simulink model "ModelPlant_DP_v3"  (R2015a)
settings: Solver=ode3  StartTime=0.0  StopTime=Simulation_Time  FixedStep=0.01  RelTol=1e-3
values from neighbouring files (symbols this model uses):
  DesiredPath = 0    [Innput.m]    (also in Input_v3.m = 1)
  Elipscenter_radi = [6 5;0 3 ]    [Innput.m]    (also in Input_v3.m)
  eta_dot_ini = [7;0;0]    [Innput.m]    (also in Input_v3.m)
  K = [2;10]    [Input_v3.m]
  K1 = diag([1,1,4])    [Input_v3.m]
  K2 = diag([200,50,3])    [Input_v3.m]    (also in inputDPgains.m = [1 0 0; 0 1 0; 0 0 1])
  l1 = [1 0 0;0 1 0;0 0 0.05]    [Input_v3.m]    (also in inputDPgains.m = [1 0 0; 0 1 0; 0 0 0.05])
  l2 = [1 0 0;0 1 0;0 0 0.05]    [Input_v3.m]    (also in inputDPgains.m = [1 0 0; 0 1 0; 0 0 0.05])
  l3 = [1 0 0;0 1 0;0 0 0.05]    [Input_v3.m]    (also in inputDPgains.m = [1 0 0; 0 1 0; 0 0 0.05])
  L_1 = 0.1    [Input_v3.m]
  L_2 = 2    [Input_v3.m]
  L_3 = 0.01    [Input_v3.m]
  LAW = 1    [Innput.m]    (also in Input_v3.m = 0)
  lim = [1.00;-20;6.45/2;-6.45/2]    [Innput.m]    (also in Input_v3.m = [20;-20;9;-9])
  lim_2 = [1.5;-22;7;-7]    [Innput.m]    (also in Input_v3.m = [25;-25;10;-10])
  m = 14.79    [Input_v3.m]    (also in ctrl_student_init.m)
  mu = mu(1)    [Innput.m]    (also in Input_v3.m = mu(2))
  pd = [2 10;0 4]    [Input_v3.m]
  T_initialDP = T_initialDP*100    (= 0)    [Input_v3.m]
  U_ref = 0.1    [Innput.m]    (also in Input_v3.m)
(part 2 of 2)

== matlab function ModelPlant_DP_v3/Subsystem1/PathParameterization/PathGenerization_Ellips/parameter generator/UpdateLaw ==
  data: s_dot output; p_d_sdot input; U_ref input; U_s output; V_1s input; mu input; eta_ds input; LAW input
function [s_dot,U_s ]= fcn(p_d_sdot,U_ref,V_1s,mu,eta_ds,LAW)


U_s=U_ref/(sqrt(p_d_sdot(1)^2+p_d_sdot(2)^2));
if LAW ==1

        s_dot=U_s-mu*V_1s;
else
        s_dot=U_s-mu/(sqrt(eta_ds(1)^2+eta_ds(2)^2))*V_1s;
end


end

== matlab function ModelPlant_DP_v3/Subsystem1/PathParameterization/PathGenerization_Straight/Path parametization /Subsystem/MATLAB Function ==
  data: InitPosOut output; DesPos input; s_in input; U_ref input; N_iteration input; N_in input; DesPosOut output; SwitchSignal_out output; N_out output; U output; s_out output; Start_time input; init_time output; flag output
function [InitPosOut,DesPosOut,SwitchSignal_out,N_out,U,s_out,init_time,flag]= fcn(DesPos,s_in,U_ref,N_iteration,N_in,Start_time)
[a,b]=size(DesPos);
N_max=b-1;
    init_time=zeros(2,1);
    init_time(1)=Start_time(1)+1;
    init_time(2)=Start_time(2);
   
if flag==2
            N_out=N_in;
            InitPosOut=DesPos(:,N_out);
            DesPosOut=DesPos(:,N_out+1);
            SwitchSignal_out=1;
            s_out=1;
            DP=1;
            flag=2;
else
    
    
if init_time(1)<N_iteration         % DP for N_iterations
    N_out=N_in;
    InitPosOut=DesPos(:,N_out);
    DesPosOut=DesPos(:,N_out+1);
    SwitchSignal_out=1;
    s_out=0;
    DP=1;
    flag=1;
    
else
    if N_in==N_max                  % if we are at final stretch
        if  s_in>=0.9999
            N_out=N_in;
            InitPosOut=DesPos(:,N_out);
            DesPosOut=DesPos(:,N_out+1);
            SwitchSignal_out=1;
            s_out=1;
            DP=1;
            flag=2;
            
        else
            N_out=N_in;
            InitPosOut=DesPos(:,N_in);
            DesPosOut=DesPos(:,N_in+1);
            SwitchSignal_out=1;
            s_out=s_in;
            DP=0;
            flag=3;
            
        end
    else
       if s_in>=0.9999
           if N_in+1 ==N_max
               SwitchSignal_out=0;
               flag=40;
           else
               SwitchSignal_out=0;
               flag=50;
           end
            N_out=N_in+1;
            InitPosOut=DesPos(:,N_out);
            DesPosOut=DesPos(:,N_out+1);
            s_out=1;
            DP=0;

       else 
            if init_time(2)==0;
                init_time(2)=1;
                SwitchSignal_out=0;
                flag=5.75;
            else
                SwitchSignal_out=1;
                flag=5.25;
            end
            N_out=N_in;
            InitPosOut=DesPos(:,N_in);
            DesPosOut=DesPos(:,N_in+1);
            s_out=s_in;
            DP=0;
            
        end
    end
    
end   
if DP==1
    U=0;
else
    U=U_ref*(1.01+ sin(2*pi*s_out-pi/2));
end

end
end

== matlab function ModelPlant_DP_v3/Subsystem1/PathParameterization/PathGenerization_Straight/parameter generator/MATLAB Function1 ==
  data: SwitchSignal_In input; SwitchSignal_Out output
function SwitchSignal_Out = fcn(SwitchSignal_In)

if SwitchSignal_In==0
    SwitchSignal_Out=1;
else
    SwitchSignal_Out=0;
end
    
end

== matlab function ModelPlant_DP_v3/Subsystem1/PathParameterization/PathGenerization_Straight/parameter generator/UpdateLaw ==
  data: s_dot output; p_d_sdot input; U_ref input; U_s output; V_1s input; mu input; eta_ds input; LAW input
function [s_dot,U_s ]= fcn(p_d_sdot,U_ref,V_1s,mu,eta_ds,LAW)


U_s=U_ref/(sqrt(p_d_sdot(1)^2+p_d_sdot(2)^2));
if LAW ==1

        s_dot=U_s-mu*V_1s;
else
        s_dot=U_s-mu/(sqrt(eta_ds(1)^2+eta_ds(2)^2))*V_1s;
end


end

== matlab function ModelPlant_DP_v3/DPObserver1/Bias/bHatDot ==
  data: bHatDot output; L3 input; eta input; etaHat input
function bHatDot = fcn(L3,eta,etaHat)

bHatDot=L3*(eta-etaHat);
%bHatDot=[0;0;0];

end

== matlab function ModelPlant_DP_v3/DPObserver1/D ==
  data: D output; etaHatDot input
function D = fcn(etaHatDot)

u=etaHatDot(1);     %u=0; 
v=etaHatDot(2);     %v=0; 
r=etaHatDot(3);     %r=0;

Xu=-0.6555;
Xuu=0.3545;
Xuuu=-3.787;
Yv=-1.33;
Yvv=-2.776;
Yvvv=-64.91;
Yr=-7.25;
Yrr=-3.45;
Yrrr=0;
Yrv=-0.805;
Yvr=-0.845;
Nv=0;
Nvv=-0.2088;
Nvvv=0;
Nr=-1.9;
Nrr=-0.75;
Nrrr=0;
Nrv=0.13;
Nvr=0.08;

d11=-Xu-Xuu*abs(u)-Xuuu*u^2;
d22=-Yv-Yvv*abs(v)-Yvvv*v^2-Yrv*abs(r);
d23=-Yr-Yvr*abs(v)-Yrr*abs(r)-Yrrr*r^2;
d32=-Nv-Nvv*abs(v)-Nvvv*v^2-Nrv*abs(r);
d33=-Nr-Nvr*abs(v)-Nrr*abs(r)-Nrrr*r^2;

D=[d11 0 0; 0 d22 d23; 0 d32 d33];

end

== matlab function ModelPlant_DP_v3/DPObserver1/Subsystem/M ==
  data: M output
function M = void

m=14.79;
M=[m+2 0 0; 0 m+10 m*0.0375; 0 m*0.0375 1.76+1];

end

== matlab function ModelPlant_DP_v3/DPObserver1/Subsystem/nuHatDot ==
  data: nuHat input; bHat input; D input; M input; L2 input; tau input; eta input; R input; etaHat input; nuHatDot output
function nuHatDot = fcn(nuHat,bHat,D,M,L2,tau,eta,R,etaHat)

%nuHatDot=inv(M)*(-D*nuHat+transpose(R)*bHat+tau+K2*transpose(R)*L2*(eta-etaHat));

nuHatDot=inv(M)*(-D*nuHat+transpose(R)*bHat+tau+transpose(R)*L2*(eta-etaHat));

end

== matlab function ModelPlant_DP_v3/DPObserver1/calcR(psi)  ==
  data: psi input; R output
function R = fcn(psi)

R=[cos(psi) -sin(psi) 0; sin(psi) cos(psi) 0; 0 0 1];

end

== matlab function ModelPlant_DP_v3/DPObserver1/etaHat/etaHatDot ==
  data: etaHat input; nuHat input; L1 input; eta input; R input; etaHatDot output
function etaHatDot = fcn(etaHat,nuHat,L1,eta,R)

%etaHatDot=zeros(3,1);
etaHatDot=R*nuHat+L1*(eta-etaHat);

end
